simulink model "SF103A_MotorReferenceModel_v001B_MappedToEA4"  (R2013b)
settings: Solver=FixedStepDiscrete  StartTime=0.0  StopTime=10.0  RelTol=1e-3
InitFcn:
  | SF103A_MotorReferenceModel_v001X_Parameters;
undefined symbols (not defined in the file or in its folder): D_DTSCLMAX_ULS, D_DTSCLMIN_ULS, D_VECUMAX_VOLTS, D_VECUMIN_VOLTS, MtrCtrl_d_Ts_slow_s, MtrCtrl_e_KeNom_VpRadpS, MtrCtrl_e_RmNom_Ohm, MtrCtrl_k_deadtimeVScale_Uls, MtrCtrl_k_FeedbackControlDisable_Cnt, MtrCtrl_k_IdBoostGain_Uls, MtrCtrl_k_IdBoostVRThreshScl_Uls, MtrCtrl_k_IdqRefIminTol_Uls, MtrCtrl_k_IdqRefTrqTol_Uls, MtrCtrl_k_LdNom_Henry, MtrCtrl_k_LqNom_Henry, MtrCtrl_k_MtrCurrDaxMaxValScl_Per, MtrCtrl_k_MtrVoltDervFiltTimeConst_Sec, MtrCtrl_k_NoofPoles_Uls, MtrCtrl_k_VoltModeDynCompEnable_Cnt, MtrCtrl_t_IdBoostTrqCharSclY_Uls, MtrCtrl_t_IdBoostTrqCmdX_MtrNm, MtrCtrl_t_IdqRefDeltaPoints_Rad, MtrCtrl_t_Q13VltgSchedXTbl_MtrRadpS, MtrCtrl_t_Q13VltgSchedYTbl_Volt, MtrCtrl_t_Q24VltgSchedXTbl_MtrRadpS, MtrCtrl_t_Q24VltgSchedYTbl_Volt
undefined symbols (not defined in the file): MtrCtrl_k_MtrVelFiltFFKn_Hz
libraries: simulink x6
(part 1 of 2)
settings Model: Creator=SZJ6LD  LastModifiedBy=lzz0tm

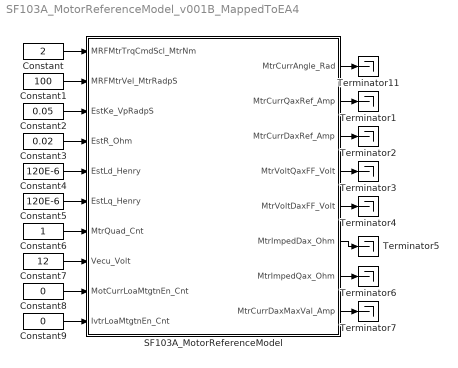
== system SF103A_MotorReferenceModel_v001B_MappedToEA4 ==
  Constant : Constant  Value=2
  Constant1 : Constant  Value=100
  Constant2 : Constant  Value=0.05
  Constant3 : Constant  Value=0.02
  Constant4 : Constant  Value=120E-6
  Constant5 : Constant  Value=120E-6
  Constant6 : Constant
  Constant7 : Constant  Value=12
  Constant8 : Constant  Value=0
  Constant9 : Constant  Value=0
  SF103A_MotorReferenceModel : Subsystem
      settings: AttributesFormatString=%<LibraryVersion>
  Terminator{1..7,11} (8 alike) : Terminator
  wires:
  SF103A_MotorReferenceModel/1(MtrCurrAngle_Rad) -> Terminator11/1
  SF103A_MotorReferenceModel/8(MtrCurrDaxMaxVal_Amp) -> Terminator7/1
  SF103A_MotorReferenceModel/7(MtrImpedQax_Ohm) -> Terminator6/1
  SF103A_MotorReferenceModel/6(MtrImpedDax_Ohm) -> Terminator5/1
  SF103A_MotorReferenceModel/5(MtrVoltDaxFF_Volt) -> Terminator4/1
  SF103A_MotorReferenceModel/4(MtrVoltQaxFF_Volt) -> Terminator3/1
  SF103A_MotorReferenceModel/3(MtrCurrDaxRef_Amp) -> Terminator2/1
  SF103A_MotorReferenceModel/2(MtrCurrQaxRef_Amp) -> Terminator1/1
  Constant/1 -> SF103A_MotorReferenceModel/1(MRFMtrTrqCmdScl_MtrNm)
  Constant1/1 -> SF103A_MotorReferenceModel/2(MRFMtrVel_MtrRadpS)
  Constant2/1 -> SF103A_MotorReferenceModel/3(EstKe_VpRadpS)
  Constant3/1 -> SF103A_MotorReferenceModel/4(EstR_Ohm)
  Constant4/1 -> SF103A_MotorReferenceModel/5(EstLd_Henry)
  Constant5/1 -> SF103A_MotorReferenceModel/6(EstLq_Henry)
  Constant6/1 -> SF103A_MotorReferenceModel/7(MtrQuad_Cnt)
  Constant7/1 -> SF103A_MotorReferenceModel/8(Vecu_Volt)
  Constant8/1 -> SF103A_MotorReferenceModel/9(MotCurrLoaMtgtnEn_Cnt)
  Constant9/1 -> SF103A_MotorReferenceModel/10(IvtrLoaMtgtnEn_Cnt)

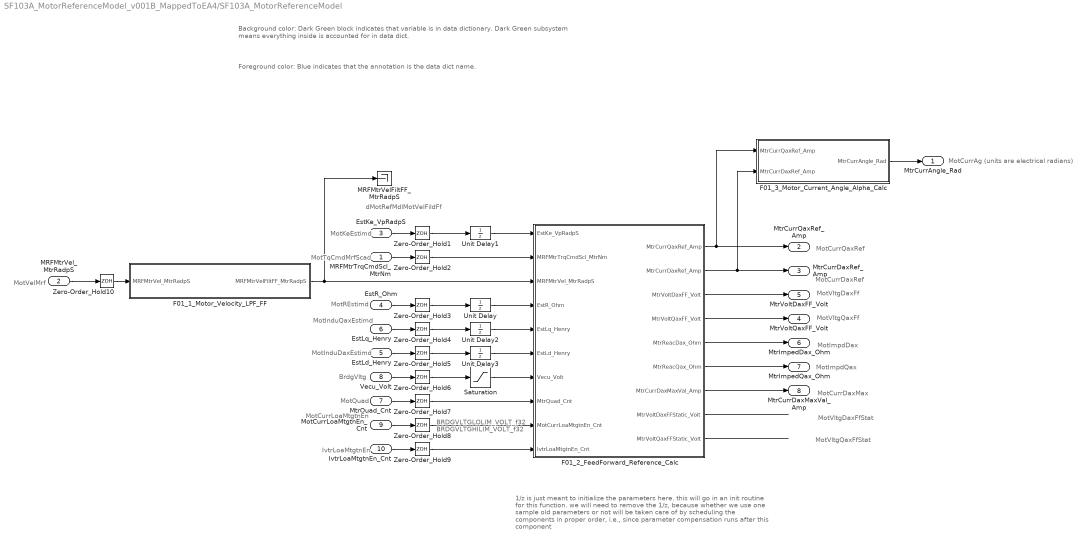
== system SF103A_MotorReferenceModel_v001B_MappedToEA4/SF103A_MotorReferenceModel ==
  note: MotVltgQaxFfStat
  note: MotVltgQaxFf
  note: MotVltgDaxFfStat
  note: MotVltgDaxFf
  note: MotImpdQax
  note: MotImpdDax
  note: MotCurrQaxRef
  note: MotCurrDaxRef
  note: MotCurrDaxMax
  note: MotCurrAg (units are electrical radians)
  note: dMotRefMdlMotVelFildFf
  note: BRDGVLTGLOLIM_VOLT_f32
      | BRDGVLTGHILIM_VOLT_f32
  note: 1/z is just meant to initialize the parameters here.
      | this will go in an init routine for this function.
      |
      | we will need to remove the 1/z, because whether we use one sample old
      | parameters or not will be taken care of by scheduling the components in
      | proper order, i.e., since parameter compensation runs after this component
  note: MotVelMrf
  note: MotTqCmdMrfScad
  note: MotREstimd
  note: MotQuad
  note: MotKeEstimd
  note: MotInduQaxEstimd
  note: MotInduDaxEstimd
  note: MotCurrLoaMtgtnEn
  note: IvtrLoaMtgtnEn
  note: BrdgVltg
  note: Background color:  Dark Green block indicates that variable is in data dictionary.
      |                                Dark Green subsystem means everything inside is accounted for in data dict.
  note: Foreground color: Blue indicates that the annotation is the data dict name.
  MRFMtrTrqCmdScl_MtrNm : Inport
  MRFMtrVel_MtrRadpS : Inport  Port=2
  EstKe_VpRadpS : Inport  Port=3
  EstR_Ohm : Inport  Port=4
  EstLd_Henry : Inport  Port=5
  EstLq_Henry : Inport  Port=6
  MtrQuad_Cnt : Inport  Port=7
  Vecu_Volt : Inport  Port=8
  MotCurrLoaMtgtnEn_Cnt : Inport  Port=9
  IvtrLoaMtgtnEn_Cnt : Inport  Port=10
  F01_1_Motor_Velocity_LPF_FF : Subsystem
  F01_2_FeedForward_Reference_Calc : Subsystem
  F01_3_Motor_Current_Angle_Alpha_Calc : Subsystem
  MRFMtrVelFiltFF_MtrRadpS : Terminator
  "Saturation  " : Saturate  UpperLimit=D_VECUMAX_VOLTS  LowerLimit=D_VECUMIN_VOLTS
      settings: AttributesFormatString=%<LowerLimit>\n%<UpperLimit>
  Unit Delay : UnitDelay  InitialCondition=MtrCtrl_e_RmNom_Ohm  SampleTime=MtrCtrl_d_Ts_slow_s
      settings: AttributesFormatString=Initial Value:\n%<X0>
  Unit Delay1 : UnitDelay  InitialCondition=MtrCtrl_e_KeNom_VpRadpS  SampleTime=MtrCtrl_d_Ts_slow_s
      settings: AttributesFormatString=Initial Value:\n%<X0>
  Unit Delay2 : UnitDelay  InitialCondition=MtrCtrl_k_LqNom_Henry  SampleTime=MtrCtrl_d_Ts_slow_s
      settings: AttributesFormatString=Initial Value:\n%<X0>
  Unit Delay3 : UnitDelay  InitialCondition=MtrCtrl_k_LdNom_Henry  SampleTime=MtrCtrl_d_Ts_slow_s
      settings: AttributesFormatString=Initial Value:\n%<X0>
  Zero-Order_Hold{1..10} (10 alike) : ZeroOrderHold  SampleTime=MtrCtrl_d_Ts_slow_s
  MtrCurrAngle_Rad : Outport
  MtrCurrQaxRef_Amp : Outport  Port=2
  MtrCurrDaxRef_Amp : Outport  Port=3
  MtrVoltQaxFF_Volt : Outport  Port=4
  MtrVoltDaxFF_Volt : Outport  Port=5
  MtrImpedDax_Ohm : Outport  Port=6
  MtrImpedQax_Ohm : Outport  Port=7
  MtrCurrDaxMaxVal_Amp : Outport  Port=8
  wires:
  F01_2_FeedForward_Reference_Calc/4(MtrVoltQaxFF_Volt) -> MtrVoltQaxFF_Volt/1
  F01_2_FeedForward_Reference_Calc/3(MtrVoltDaxFF_Volt) -> MtrVoltDaxFF_Volt/1
  F01_2_FeedForward_Reference_Calc/5(MtrReacDax_Ohm) -> MtrImpedDax_Ohm/1
  F01_2_FeedForward_Reference_Calc/6(MtrReacQax_Ohm) -> MtrImpedQax_Ohm/1
  MtrQuad_Cnt/1 -> Zero-Order_Hold7/1
  Vecu_Volt/1 -> Zero-Order_Hold6/1
  F01_3_Motor_Current_Angle_Alpha_Calc/1(MtrCurrAngle_Rad) -> MtrCurrAngle_Rad/1
  MRFMtrTrqCmdScl_MtrNm/1 -> Zero-Order_Hold2/1
  EstLq_Henry/1 -> Zero-Order_Hold4/1
  EstLd_Henry/1 -> Zero-Order_Hold5/1
  EstR_Ohm/1 -> Zero-Order_Hold3/1
  EstKe_VpRadpS/1 -> Zero-Order_Hold1/1
  F01_1_Motor_Velocity_LPF_FF/1(MRFMtrVelFiltFF_MtrRadpS) -> F01_2_FeedForward_Reference_Calc/3(MRFMtrVel_MtrRadpS), MRFMtrVelFiltFF_MtrRadpS/1
  MRFMtrVel_MtrRadpS/1 -> Zero-Order_Hold10/1
  F01_2_FeedForward_Reference_Calc/7(MtrCurrDaxMaxVal_Amp) -> MtrCurrDaxMaxVal_Amp/1
  F01_2_FeedForward_Reference_Calc/9(MtrVoltQaxFFStatic_Volt) -> ?
  F01_2_FeedForward_Reference_Calc/8(MtrVoltDaxFFStatic_Volt) -> ?
  MotCurrLoaMtgtnEn_Cnt/1 -> Zero-Order_Hold8/1
  F01_2_FeedForward_Reference_Calc/1(MtrCurrQaxRef_Amp) -> F01_3_Motor_Current_Angle_Alpha_Calc/1(MtrCurrQaxRef_Amp), MtrCurrQaxRef_Amp/1
  F01_2_FeedForward_Reference_Calc/2(MtrCurrDaxRef_Amp) -> F01_3_Motor_Current_Angle_Alpha_Calc/2(MtrCurrDaxRef_Amp), MtrCurrDaxRef_Amp/1
  Unit Delay/1 -> F01_2_FeedForward_Reference_Calc/4(EstR_Ohm)
  Unit Delay1/1 -> F01_2_FeedForward_Reference_Calc/1(EstKe_VpRadpS)
  Unit Delay2/1 -> F01_2_FeedForward_Reference_Calc/5(EstLq_Henry)
  Unit Delay3/1 -> F01_2_FeedForward_Reference_Calc/6(EstLd_Henry)
  Zero-Order_Hold10/1 -> F01_1_Motor_Velocity_LPF_FF/1(MRFMtrVel_MtrRadpS)
  Zero-Order_Hold1/1 -> Unit Delay1/1
  Zero-Order_Hold2/1 -> F01_2_FeedForward_Reference_Calc/2(MRFMtrTrqCmdScl_MtrNm)
  Zero-Order_Hold3/1 -> Unit Delay/1
  Zero-Order_Hold4/1 -> Unit Delay2/1
  Zero-Order_Hold5/1 -> Unit Delay3/1
  Zero-Order_Hold6/1 -> "Saturation  "/1
  Zero-Order_Hold7/1 -> F01_2_FeedForward_Reference_Calc/8(MtrQuad_Cnt)
  Zero-Order_Hold8/1 -> F01_2_FeedForward_Reference_Calc/9(MotCurrLoaMtgtnEn_Cnt)
  "Saturation  "/1 -> F01_2_FeedForward_Reference_Calc/7(Vecu_Volt)
  IvtrLoaMtgtnEn_Cnt/1 -> Zero-Order_Hold9/1
  Zero-Order_Hold9/1 -> F01_2_FeedForward_Reference_Calc/10(IvtrLoaMtgtnEn_Cnt)

== system SF103A_MotorReferenceModel_v001B_MappedToEA4/SF103A_MotorReferenceModel/F01_1_Motor_Velocity_LPF_FF ==
  note: MotRefMdlMotVelLpFiltFrq
  MRFMtrVel_MtrRadpS : Inport
  1LP1-CF Filter : Subsystem  mask{Ts=MtrCtrl_d_Ts_slow_s, Kn_Hz=MtrCtrl_k_MtrVelFiltFFKn_Hz, IC=0}
      mask prompts: Ts "Function Time Step (seconds)"; Kn_Hz "Cutoff Frequency in Hz"; IC "Initial Condition (Enineering Units)"
      mask init:
      | %Convert cutoff frequency from Hz into floating point "counts"
      | Kn_Cnt = 1-exp(-2*pi*Kn_Hz*Ts);
      | 
      | %Filter design document originally called this value Knum
      | Knum = Kn_Cnt;
      settings: AttributesFormatString=%<Kn_Hz>
      mask Display:
      | a = [2:0.1:5.2]';
      | b = sin(2*a);
      | c = 0.7*sin(25*a);
      | d = b+c;
      | e = vertcat(d, b);
      | plot(e);
  MRFMtrVelFiltFF_MtrRadpS : Outport
  wires:
  MRFMtrVel_MtrRadpS/1 -> 1LP1-CF Filter/1(In1)
  1LP1-CF Filter/1(Out) -> MRFMtrVelFiltFF_MtrRadpS/1

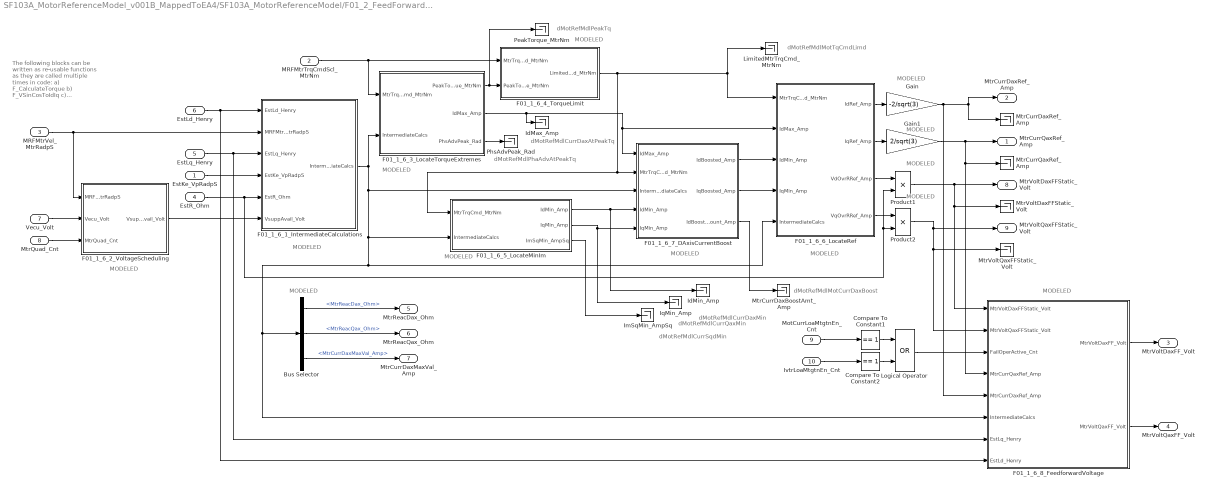
== system SF103A_MotorReferenceModel_v001B_MappedToEA4/SF103A_MotorReferenceModel/F01_2_FeedForward_Reference_Calc ==
  note: MODELED
  note: dMotRefMdlMotCurrDaxBoost
  note: dMotRefMdlCurrSqdMin
  note: dMotRefMdlCurrQaxMin
  note: dMotRefMdlCurrDaxMin
  note: dMotRefMdlCurrDaxAtPeakTq
  note: dMotRefMdlPhaAdvAtPeakTq
  note: dMotRefMdlPeakTq
  note: dMotRefMdlMotTqCmdLimd
  note: The following blocks can be written as re-usable functions
      | as they are called multiple times in code:
      | a) F_CalculateTorque
      | b)  F_VSinCosToIdIq
      | c) F_ParabolicInterpolation
      | d) F_CalcIqCommand
      | e) F_ImVSIdq
      | f) F_ItoV
      | g) F_VoltTest
  note: MODELED
  note: MODELED
  note: MODELED
  note: MODELED
  note: MODELED
  note: MODELED
  note: MODELED
  note: MODELED
  note: MODELED
  note: MODELED
  note: MODELED
  note: MODELED
  EstKe_VpRadpS : Inport
  MRFMtrTrqCmdScl_MtrNm : Inport  Port=2
  MRFMtrVel_MtrRadpS : Inport  Port=3
  EstR_Ohm : Inport  Port=4
  EstLq_Henry : Inport  Port=5
  EstLd_Henry : Inport  Port=6
  Vecu_Volt : Inport  Port=7
  MtrQuad_Cnt : Inport  Port=8
  MotCurrLoaMtgtnEn_Cnt : Inport  Port=9
  IvtrLoaMtgtnEn_Cnt : Inport  Port=10
  Bus Selector : BusSelector  OutputSignals=MtrReacDax_Ohm,MtrReacQax_Ohm,MtrCurrDaxMaxVal_Amp
  Compare To Constant1 : simulink/Logic and Bit Operations/Compare To Constant  relop===  const=1  OutDataTypeStr=uint8
  Compare To Constant2 : simulink/Logic and Bit Operations/Compare To Constant  relop===  const=1  OutDataTypeStr=uint8
  F01_1_6_1_IntermediateCalculations : Subsystem
  F01_1_6_2_VoltageScheduling : Subsystem
  F01_1_6_3_LocateTorqueExtremes : Subsystem
  F01_1_6_4_TorqueLimit : Subsystem
  F01_1_6_5_LocateMinIm : Subsystem
  F01_1_6_6_LocateRef : Subsystem
  F01_1_6_7_DAxisCurrentBoost : Subsystem
  F01_1_6_8_FeedforwardVoltage : Subsystem
  Gain : Gain  Gain=-2/sqrt(3)
  Gain1 : Gain  Gain=2/sqrt(3)
  IdMax_Amp : Terminator
  IdMin_Amp : Terminator
  ImSqMin_AmpSq : Terminator
  IqMin_Amp : Terminator
  "LimitedMtrTrqCmd_MtrNm " : Terminator
  Logical Operator : Logic  Operator=OR  AllPortsSameDT=off  OutDataTypeStr=boolean
  MtrCurrDaxBoostAmt_Amp : Terminator
  "MtrCurrDaxRef_Amp " : Terminator
  "MtrCurrQaxRef_Amp " : Terminator
  "MtrVoltDaxFFStatic_Volt " : Terminator
  "MtrVoltQaxFFStatic_Volt " : Terminator
  PeakTorque_MtrNm : Terminator
  PhsAdvPeak_Rad : Terminator
  Product1 : Product  RndMeth=Zero
  Product2 : Product  RndMeth=Zero
  MtrCurrQaxRef_Amp : Outport
  MtrCurrDaxRef_Amp : Outport  Port=2
  MtrVoltDaxFF_Volt : Outport  Port=3
  MtrVoltQaxFF_Volt : Outport  Port=4
  MtrReacDax_Ohm : Outport  Port=5
  MtrReacQax_Ohm : Outport  Port=6
  MtrCurrDaxMaxVal_Amp : Outport  Port=7
  MtrVoltDaxFFStatic_Volt : Outport  Port=8
  MtrVoltQaxFFStatic_Volt : Outport  Port=9
  wires:
  Gain/1 -> F01_1_6_8_FeedforwardVoltage/5(MtrCurrDaxRef_Amp), MtrCurrDaxRef_Amp/1, "MtrCurrDaxRef_Amp "/1
  Product2/1 -> F01_1_6_8_FeedforwardVoltage/2(MtrVoltQaxFFStatic_Volt), "MtrVoltQaxFFStatic_Volt "/1, MtrVoltQaxFFStatic_Volt/1
  Product1/1 -> F01_1_6_8_FeedforwardVoltage/1(MtrVoltDaxFFStatic_Volt), "MtrVoltDaxFFStatic_Volt "/1, MtrVoltDaxFFStatic_Volt/1
  Gain1/1 -> F01_1_6_8_FeedforwardVoltage/4(MtrCurrQaxRef_Amp), "MtrCurrQaxRef_Amp "/1, MtrCurrQaxRef_Amp/1
  F01_1_6_8_FeedforwardVoltage/2(MtrVoltQaxFF_Volt) -> MtrVoltQaxFF_Volt/1
  F01_1_6_8_FeedforwardVoltage/1(MtrVoltDaxFF_Volt) -> MtrVoltDaxFF_Volt/1
  Bus Selector/1 -> MtrReacDax_Ohm/1  "<MtrReacDax_Ohm>"
  Bus Selector/2 -> MtrReacQax_Ohm/1  "<MtrReacQax_Ohm>"
  F01_1_6_7_DAxisCurrentBoost/3(IdBoostAmount_Amp) -> MtrCurrDaxBoostAmt_Amp/1
  F01_1_6_7_DAxisCurrentBoost/2(IqBoosted_Amp) -> F01_1_6_6_LocateRef/4(IqMin_Amp)
  F01_1_6_7_DAxisCurrentBoost/1(IdBoosted_Amp) -> F01_1_6_6_LocateRef/3(IdMin_Amp)
  MtrQuad_Cnt/1 -> F01_1_6_2_VoltageScheduling/3(MtrQuad_Cnt)
  Vecu_Volt/1 -> F01_1_6_2_VoltageScheduling/2(Vecu_Volt)
  F01_1_6_2_VoltageScheduling/1(VsuppAvail_Volt) -> F01_1_6_1_IntermediateCalculations/6(VsuppAvail_Volt)
  F01_1_6_6_LocateRef/4(VqOvrRRef_Amp) -> Product2/1
  F01_1_6_6_LocateRef/3(VdOvrRRef_Amp) -> Product1/1
  F01_1_6_6_LocateRef/2(IqRef_Amp) -> Gain1/1
  F01_1_6_6_LocateRef/1(IdRef_Amp) -> Gain/1
  F01_1_6_5_LocateMinIm/3(ImSqMin_AmpSq) -> ImSqMin_AmpSq/1
  F01_1_6_3_LocateTorqueExtremes/3(PhsAdvPeak_Rad) -> PhsAdvPeak_Rad/1
  F01_1_6_5_LocateMinIm/2(IqMin_Amp) -> F01_1_6_7_DAxisCurrentBoost/5(IqMin_Amp), IqMin_Amp/1
  F01_1_6_5_LocateMinIm/1(IdMin_Amp) -> F01_1_6_7_DAxisCurrentBoost/4(IdMin_Amp), IdMin_Amp/1
  F01_1_6_3_LocateTorqueExtremes/2(IdMax_Amp) -> F01_1_6_7_DAxisCurrentBoost/1(IdMax_Amp), F01_1_6_6_LocateRef/2(IdMax_Amp), IdMax_Amp/1
  MRFMtrTrqCmdScl_MtrNm/1 -> F01_1_6_3_LocateTorqueExtremes/1(MtrTrqCmd_MtrNm), F01_1_6_4_TorqueLimit/1(MtrTrqCmd_MtrNm)
  F01_1_6_3_LocateTorqueExtremes/1(PeakTorque_MtrNm) -> PeakTorque_MtrNm/1, F01_1_6_4_TorqueLimit/2(PeakTorque_MtrNm)
  EstR_Ohm/1 -> Product2/2, Product1/2, F01_1_6_1_IntermediateCalculations/5(EstR_Ohm)
  EstKe_VpRadpS/1 -> F01_1_6_1_IntermediateCalculations/4(EstKe_VpRadpS)
  MRFMtrVel_MtrRadpS/1 -> F01_1_6_2_VoltageScheduling/1(MRFMtrVel_MtrRadpS), F01_1_6_1_IntermediateCalculations/2(MRFMtrVel_MtrRadpS)
  EstLd_Henry/1 -> F01_1_6_1_IntermediateCalculations/1(EstLd_Henry), F01_1_6_8_FeedforwardVoltage/8(EstLd_Henry)
  F01_1_6_1_IntermediateCalculations/1(IntermediateCalcs) -> F01_1_6_7_DAxisCurrentBoost/3(IntermediateCalcs), F01_1_6_5_LocateMinIm/2(IntermediateCalcs), F01_1_6_6_LocateRef/5(IntermediateCalcs), F01_1_6_8_FeedforwardVoltage/6(IntermediateCalcs), Bus Selector/1, F01_1_6_3_LocateTorqueExtremes/2(IntermediateCalcs)
  F01_1_6_4_TorqueLimit/1(LimitedMtrTrqCmd_MtrNm) -> F01_1_6_5_LocateMinIm/1(MtrTrqCmd_MtrNm), F01_1_6_7_DAxisCurrentBoost/2(MtrTrqCmd_MtrNm), "LimitedMtrTrqCmd_MtrNm "/1, F01_1_6_6_LocateRef/1(MtrTrqCmd_MtrNm)
  Compare To Constant1/1 -> Logical Operator/1
  EstLq_Henry/1 -> F01_1_6_8_FeedforwardVoltage/7(EstLq_Henry), F01_1_6_1_IntermediateCalculations/3(EstLq_Henry)
  Bus Selector/3 -> MtrCurrDaxMaxVal_Amp/1  "<MtrCurrDaxMaxVal_Amp>"
  Compare To Constant2/1 -> Logical Operator/2
  Logical Operator/1 -> F01_1_6_8_FeedforwardVoltage/3(FailOperActive_Cnt)
  MotCurrLoaMtgtnEn_Cnt/1 -> Compare To Constant1/1
  IvtrLoaMtgtnEn_Cnt/1 -> Compare To Constant2/1

== system SF103A_MotorReferenceModel_v001B_MappedToEA4/SF103A_MotorReferenceModel/F01_3_Motor_Current_Angle_Alpha_Calc ==
  MtrCurrQaxRef_Amp : Inport
  MtrCurrDaxRef_Amp : Inport  Port=2
  atan2 : Trigonometry  Operator=atan2
  MtrCurrAngle_Rad : Outport
  wires:
  MtrCurrQaxRef_Amp/1 -> atan2/2
  MtrCurrDaxRef_Amp/1 -> atan2/1
  atan2/1 -> MtrCurrAngle_Rad/1

== system SF103A_MotorReferenceModel_v001B_MappedToEA4/SF103A_MotorReferenceModel/F01_1_Motor_Velocity_LPF_FF/1LP1-CF Filter ==
  note: Filter layout from spreadsheet
  note: This Subsystem represents a type 1LP1-CF Low-Pass filter with floating point math. Layout and nomenclature taken from Design Document authored by Mark Colosky.
  note: REVISIONS
      |   Feb 13, 2012.  Date created.
      |   Feb 17, 2012.  Conversion from Hz to Knum moved to Initialization tab of mask dialog box.
      |   Feb 20, 2012.  Parameterized 1/z block Initial Condition instead of hard-coded = 0.
  In1 : Inport
  Constant : Constant  Value=Knum  SampleTime=Ts
  Integer Delay : Delay  DelayLength=1  InitialCondition=IC  SampleTime=Ts
  Product1 : Product  RndMeth=Zero
  Sum : Sum  Inputs=|+-
  Sum1 : Sum  Inputs=|++
  Out : Outport
  wires:
  Sum1/1 -> Out/1, Integer Delay/1  "e"
  In1/1 -> Sum/1  "Unfiltered_Signal"
  Integer Delay/1 -> Sum/2, Sum1/2  "f"
  Product1/1 -> Sum1/1  "d"
  Constant/1 -> Product1/1
  Sum/1 -> Product1/2  "c"

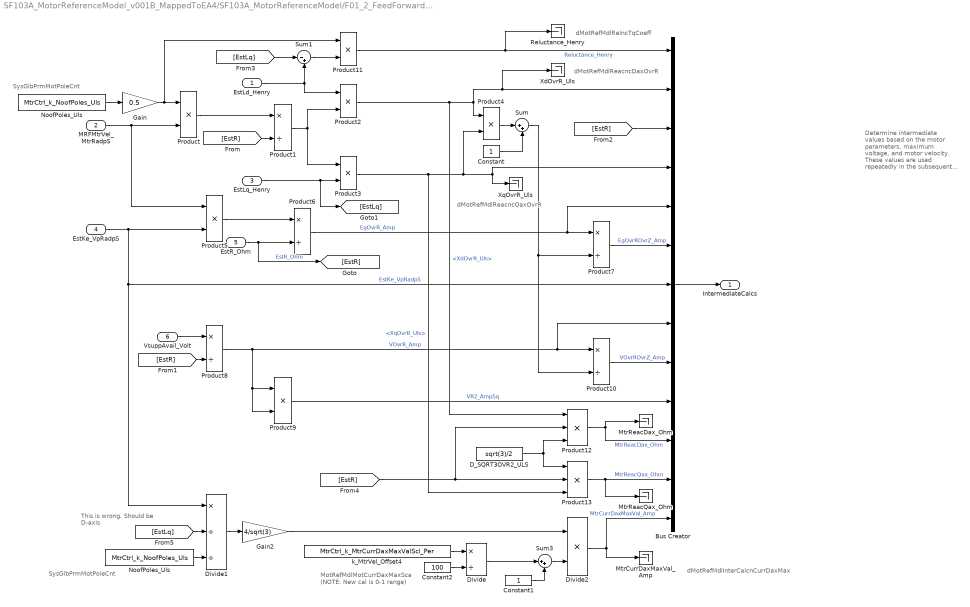
== system SF103A_MotorReferenceModel_v001B_MappedToEA4/SF103A_MotorReferenceModel/F01_2_FeedForward_Reference_Calc/F01_1_6_1_IntermediateCalculations ==
  note: This is wrong.
      | Should be D-axis
  note: MotRefMdlMotCurrDaxMaxSca
      | (NOTE:  New cal is 0-1 range)
  note: SysGlbPrmMotPoleCnt
  note: dMotRefMdlReacncDaxOvrR
  note: dMotRefMdlRelncTqCoeff
  note: dMotRefMdlInterCalcnCurrDaxMax
  note: Determine intermediate values based on the motor parameters, maximum voltage, and motor velocity.
      | These values are used repeatedly in the subsequent iterative solutions and performing these calculations once
      | in advance decreases computation time and reduces the possibility of introducing error.
  note: dMotRefMdlReacncQaxOvrR
  note: SysGlbPrmMotPoleCnt
  EstLd_Henry : Inport
  MRFMtrVel_MtrRadpS : Inport  Port=2
  EstLq_Henry : Inport  Port=3
  EstKe_VpRadpS : Inport  Port=4
  EstR_Ohm : Inport  Port=5
  VsuppAvail_Volt : Inport  Port=6
  Bus Creator : BusCreator  Inputs=13
  Constant : Constant
  Constant1 : Constant  SampleTime=MtrCtrl_d_Ts_slow_s
  Constant2 : Constant  Value=100  SampleTime=MtrCtrl_d_Ts_slow_s
  D_SQRT3OVR2_ULS : Constant  Value=sqrt(3)/2  SampleTime=MtrCtrl_d_Ts_slow_s
  Divide : Product  Inputs=*/
  Divide1 : Product  Inputs=*//
  Divide2 : Product
  Gain : Gain  Gain=0.5  SampleTime=MtrCtrl_d_Ts_slow_s
  Gain2 : Gain  Gain=4/sqrt(3)  SampleTime=MtrCtrl_d_Ts_slow_s
  "MtrCurrDaxMaxVal_Amp  " : Terminator
  "MtrReacDax_Ohm   " : Terminator
  "MtrReacQax_Ohm  " : Terminator
  NoofPoles_Uls : Constant  Value=MtrCtrl_k_NoofPoles_Uls
  "NoofPoles_Uls " : Constant  Value=MtrCtrl_k_NoofPoles_Uls
  Product : Product  SampleTime=MtrCtrl_d_Ts_slow_s  RndMeth=Zero
  Product1 : Product  Inputs=*/  RndMeth=Zero
  Product10 : Product  Inputs=*/  SampleTime=MtrCtrl_d_Ts_slow_s  RndMeth=Zero
  Product{2..4,11} (4 alike) : Product  RndMeth=Zero
  Product12 : Product  Inputs=3  RndMeth=Zero
  Product13 : Product  Inputs=3  RndMeth=Zero
  Product5 : Product  SampleTime=MtrCtrl_d_Ts_slow_s  RndMeth=Zero
  Product6 : Product  Inputs=*/  RndMeth=Zero
  Product7 : Product  Inputs=*/  SampleTime=MtrCtrl_d_Ts_slow_s  RndMeth=Zero
  Product8 : Product  Inputs=*/  SampleTime=MtrCtrl_d_Ts_slow_s  RndMeth=Zero
  Product9 : Product  SampleTime=MtrCtrl_d_Ts_slow_s  RndMeth=Zero
  Reluctance_Henry : Terminator
  Sum : Sum  Inputs=|++
  Sum1 : Sum  Inputs=|-+
  Sum3 : Sum  Inputs=|++
  XdOvrR_Uls : Terminator
  XqOvrR_Uls : Terminator
  k_MtrVel_Offset4 : Constant  Value=MtrCtrl_k_MtrCurrDaxMaxValScl_Per  SampleTime=MtrCtrl_d_Ts_slow_s
  IntermediateCalcs : Outport
  wires:
  VsuppAvail_Volt/1 -> Product8/1
  Bus Creator/1 -> IntermediateCalcs/1
  NoofPoles_Uls/1 -> Gain/1
  Product10/1 -> Bus Creator/9  "VOvrROvrZ_Amp"
  Product11/1 -> Bus Creator/1, Reluctance_Henry/1  "Reluctance_Henry"
  Sum1/1 -> Product11/2
  [EstLq] -> Sum1/1
  [EstR] -> Bus Creator/3
  Product9/1 -> Bus Creator/10  "VR2_AmpSq"
  Product8/1 -> Bus Creator/8, Product10/1, Product9/2, Product9/1  "VOvrR_Amp"
  [EstR] -> Product8/2
  Product7/1 -> Bus Creator/6  "EgOvrROvrZ_Amp"
  Product6/1 -> Bus Creator/5, Product7/1  "EgOvrR_Amp"
  [EstR] -> Product1/2
  EstR_Ohm/1 -> Product6/2, [EstR]  "EstR_Ohm"
  Product5/1 -> Product6/1
  EstKe_VpRadpS/1 -> Product5/2, Divide1/1, Bus Creator/7  "EstKe_VpRadpS"
  Sum/1 -> Product10/2, Product7/2
  Constant/1 -> Sum/2
  Product4/1 -> Sum/1
  EstLq_Henry/1 -> Product3/2, [EstLq]
  EstLd_Henry/1 -> Sum1/2, Product2/1
  Product1/1 -> Product3/1, Product2/2
  Product/1 -> Product1/1
  MRFMtrVel_MtrRadpS/1 -> Product5/1, Product/2
  Gain/1 -> Product11/1, Product/1
  D_SQRT3OVR2_ULS/1 -> Product12/3, Product13/1
  Product3/1 -> Product13/3, XqOvrR_Uls/1, Bus Creator/4, Product4/2  "<XqOvrR_Uls>"
  [EstR] -> Product12/2, Product13/2
  Product13/1 -> Bus Creator/12, "MtrReacQax_Ohm  "/1  "MtrReacQax_Ohm"
  Product12/1 -> "MtrReacDax_Ohm   "/1, Bus Creator/11  "MtrReacDax_Ohm"
  Product2/1 -> Product12/1, XdOvrR_Uls/1, Bus Creator/2, Product4/1  "<XdOvrR_Uls>"
  "NoofPoles_Uls "/1 -> Divide1/3
  Divide1/1 -> Gain2/1
  Gain2/1 -> Divide2/1
  Constant1/1 -> Sum3/2
  Divide/1 -> Sum3/1
  k_MtrVel_Offset4/1 -> Divide/1
  Constant2/1 -> Divide/2
  Sum3/1 -> Divide2/2
  Divide2/1 -> Bus Creator/13, "MtrCurrDaxMaxVal_Amp  "/1  "MtrCurrDaxMaxVal_Amp"
  [EstLq] -> Divide1/2

== system SF103A_MotorReferenceModel_v001B_MappedToEA4/SF103A_MotorReferenceModel/F01_2_FeedForward_Reference_Calc/F01_1_6_2_VoltageScheduling ==
  note: IVTRDEADTIBRDGVLTGSCALOLIM_ULS_F32
      | IVTRDEADTIBRDGVLTGSCAHILIM_ULS_F32
  note: MotRefMdlIvtrDeadTiBrdgVltgSca
  note: MotRefMdlQ13VltgSdlXTbl
      | MotRefMdlQ13VltgSdlYTbl
  note: MotRefMdlQ24VltgSdlXTbl
      | MotRefMdlQ24VltgSdlYTbl
  MRFMtrVel_MtrRadpS : Inport
  Vecu_Volt : Inport  Port=2
  MtrQuad_Cnt : Inport  Port=3
  Abs : Abs  SampleTime=MtrCtrl_d_Ts_slow_s
  Compare To Constant : simulink/Logic and Bit Operations/Compare To Constant  relop===  const=3.0  OutDataTypeStr=uint8
  Compare To Constant1 : simulink/Logic and Bit Operations/Compare To Constant  relop===  const=1  OutDataTypeStr=uint8
  Logical Operator : Logic  Operator=OR  AllPortsSameDT=off  OutDataTypeStr=boolean
  Lookup Table : Lookup  InputValues=MtrCtrl_t_Q13VltgSchedXTbl_MtrRadpS  Table=MtrCtrl_t_Q13VltgSchedYTbl_Volt  LookUpMeth=Interpolation-Use End Values
      settings: AttributesFormatString=%<InputValues>\n%<Table>
  Lookup Table1 : Lookup  InputValues=MtrCtrl_t_Q24VltgSchedXTbl_MtrRadpS  Table=MtrCtrl_t_Q24VltgSchedYTbl_Volt  LookUpMeth=Interpolation-Use End Values
      settings: AttributesFormatString=%<InputValues>\n%<Table>
  Product : Product  RndMeth=Zero
  "Saturation  " : Saturate  UpperLimit=D_DTSCLMAX_ULS  LowerLimit=D_DTSCLMIN_ULS
      settings: AttributesFormatString=%<LowerLimit>\n%<UpperLimit>
  Sum : Sum  Inputs=|+-
  Switch : Switch  Criteria=u2 > Threshold
  k_deadtimeVScale : Constant  Value=MtrCtrl_k_deadtimeVScale_Uls  SampleTime=MtrCtrl_d_Ts_slow_s
  VsuppAvail_Volt : Outport
  wires:
  Sum/1 -> VsuppAvail_Volt/1
  Switch/1 -> Sum/2
  Lookup Table1/1 -> Switch/3
  Lookup Table/1 -> Switch/1
  Logical Operator/1 -> Switch/2
  MtrQuad_Cnt/1 -> Compare To Constant1/1, Compare To Constant/1
  Compare To Constant1/1 -> Logical Operator/2
  Compare To Constant/1 -> Logical Operator/1
  Product/1 -> Sum/1
  k_deadtimeVScale/1 -> "Saturation  "/1
  Vecu_Volt/1 -> Product/1
  Abs/1 -> Lookup Table1/1, Lookup Table/1
  MRFMtrVel_MtrRadpS/1 -> Abs/1
  "Saturation  "/1 -> Product/2

== system SF103A_MotorReferenceModel_v001B_MappedToEA4/SF103A_MotorReferenceModel/F01_2_FeedForward_Reference_Calc/F01_1_6_3_LocateTorqueExtremes ==
  note: Determine the maximum possible torque and the direct axis current that corresponds to that current given the Intermediate calculation values
      |  and the sign of the torque command.  In order to do this, a series of search brackets are created by rotating the voltage vector completely around
      |  a circle in a finite number of steps.  Then the bracket array is searched for the maximum. If the resulting brackets include an angle of zero, the
      | brackets are adjusted to wrap the angle and avoid a discontinuity at zero. Finally, iterative parabolic interpolation is used to refine the
      | location of the maximum.
  note: MODELED
      | (Init runnable)
  note: MODELED
  note: MODELED
  note: MODELED
  note: MODELED
  MtrTrqCmd_MtrNm : Inport
  IntermediateCalcs : Inport  Port=2
  F01_1_6_3_1_FillBracketArrays : Subsystem
  F01_1_6_3_2_FindPeakTorques : Subsystem
  F01_1_6_3_3_ChooseDeltaBrackets : Subsystem
  F01_1_6_3_4_WrapBracketAngles : Subsystem
  F01_1_6_3_5_InterpolatePeakTorque : Subsystem
  PeakTorque_MtrNm : Outport
  IdMax_Amp : Outport  Port=2
  PhsAdvPeak_Rad : Outport  Port=3
  wires:
  MtrTrqCmd_MtrNm/1 -> F01_1_6_3_2_FindPeakTorques/2(MtrTrqCmd_MtrNm)
  F01_1_6_3_5_InterpolatePeakTorque/3(PhsAdvPeak_Rad) -> PhsAdvPeak_Rad/1
  F01_1_6_3_5_InterpolatePeakTorque/2(IdMax_Amp) -> IdMax_Amp/1
  F01_1_6_3_5_InterpolatePeakTorque/1(PeakTorque_MtrNm) -> PeakTorque_MtrNm/1
  F01_1_6_3_4_WrapBracketAngles/1(Points) -> F01_1_6_3_5_InterpolatePeakTorque/1(Points)
  F01_1_6_3_2_FindPeakTorques/1(PeakTrqIndex) -> F01_1_6_3_4_WrapBracketAngles/2(Index)
  F01_1_6_3_3_ChooseDeltaBrackets/1(Brackets) -> F01_1_6_3_4_WrapBracketAngles/1(Brackets), F01_1_6_3_2_FindPeakTorques/1(Brackets)
  F01_1_6_3_1_FillBracketArrays/1(BracketArray) -> F01_1_6_3_3_ChooseDeltaBrackets/1(BracketArray)
  IntermediateCalcs/1 -> F01_1_6_3_5_InterpolatePeakTorque/2(IntermediateCalcs), F01_1_6_3_3_ChooseDeltaBrackets/2(IntermediateCalcs)

== system SF103A_MotorReferenceModel_v001B_MappedToEA4/SF103A_MotorReferenceModel/F01_2_FeedForward_Reference_Calc/F01_1_6_4_TorqueLimit ==
  note: Limit the torque command to less than or equal to the value found in
      |  Locate Torque Extremes  to avoid searching for impossible solutions
  MtrTrqCmd_MtrNm : Inport
  PeakTorque_MtrNm : Inport  Port=2
  Sum : Sum  Inputs=|-+
  Sum1 : Sum  Inputs=+-|
  Switch : Switch
  Switch1 : Switch  Criteria=u2 > Threshold
  Switch2 : Switch
  LimitedMtrTrqCmd_MtrNm : Outport
  wires:
  Switch2/1 -> Switch/3
  Switch1/1 -> Switch/1
  Sum1/1 -> Switch2/2
  Sum/1 -> Switch1/2
  PeakTorque_MtrNm/1 -> Switch1/1, Sum/1, Switch2/3, Sum1/2
  Switch/1 -> LimitedMtrTrqCmd_MtrNm/1
  MtrTrqCmd_MtrNm/1 -> Switch2/1, Sum1/1, Switch1/3, Sum/2, Switch/2

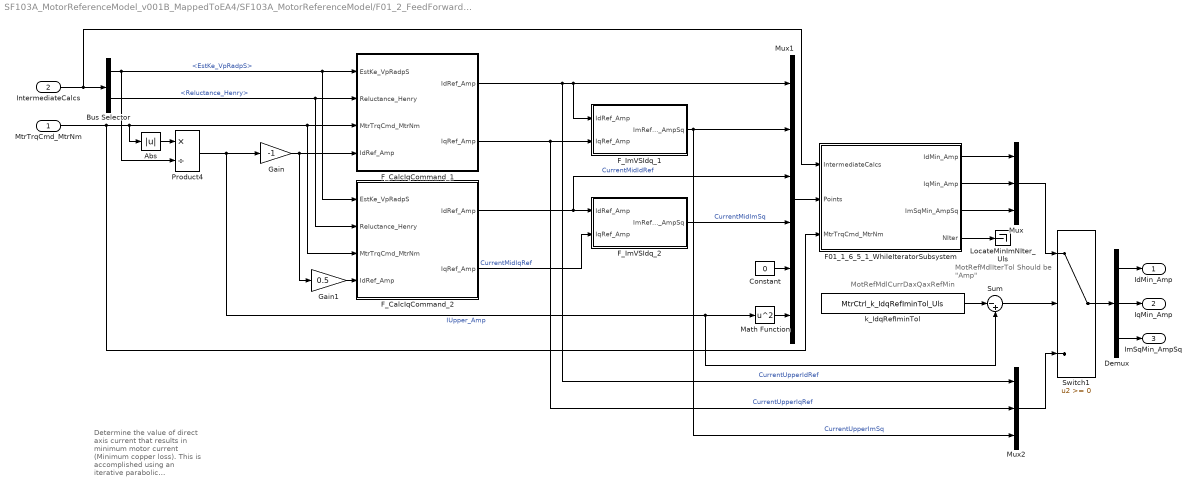
== system SF103A_MotorReferenceModel_v001B_MappedToEA4/SF103A_MotorReferenceModel/F01_2_FeedForward_Reference_Calc/F01_1_6_5_LocateMinIm ==
  note: MotRefMdlIterTol
      | Should be "Amp"
  note: MotRefMdlCurrDaxQaxRefMin
  note: Determine the value of direct axis current that results in minimum motor current (Minimum copper loss).
      | This is accomplished using an iterative parabolic interpolation. The triple of points used to initialize the
      | interpolation include:
      | a.	Direct axis current equal to zero
      | b.	Direct axis current equal to torque command divided by motor constant
      | c.	Direct axis current equal to one half of point b.
  MtrTrqCmd_MtrNm : Inport
  IntermediateCalcs : Inport  Port=2
  Abs : Abs
  Bus Selector : BusSelector  OutputSignals=EstKe_VpRadpS,Reluctance_Henry
  Constant : Constant  Value=0
  Demux : Demux  Outputs=3
  F01_1_6_5_1_WhileIteratorSubsystem : Subsystem  TreatAsAtomicUnit=on
  F_CalcIqCommand_1 : Subsystem
  F_CalcIqCommand_2 : Subsystem
  F_ImVSIdq_1 : Subsystem
  F_ImVSIdq_2 : Subsystem
  Gain : Gain  Gain=-1
  Gain1 : Gain  Gain=0.5
  LocateMinImNIter_Uls : Terminator
  Math Function : Math  Operator=square  SaturateOnIntegerOverflow=on
  Mux : Mux  Inputs=3
  Mux1 : Mux  Inputs=6
  Mux2 : Mux  Inputs=3
  Product4 : Product  Inputs=*/  RndMeth=Zero
  Sum : Sum  Inputs=|-+
  Switch1 : Switch
  k_IdqRefIminTol : Constant  Value=MtrCtrl_k_IdqRefIminTol_Uls
  IdMin_Amp : Outport
  IqMin_Amp : Outport  Port=2
  ImSqMin_AmpSq : Outport  Port=3
  wires:
  F01_1_6_5_1_WhileIteratorSubsystem/4(NIter) -> LocateMinImNIter_Uls/1
  Demux/2 -> IqMin_Amp/1
  Demux/1 -> IdMin_Amp/1
  F01_1_6_5_1_WhileIteratorSubsystem/2(IqMin_Amp) -> Mux/2
  F01_1_6_5_1_WhileIteratorSubsystem/1(IdMin_Amp) -> Mux/1
  Demux/3 -> ImSqMin_AmpSq/1
  Switch1/1 -> Demux/1
  Mux/1 -> Switch1/1
  Mux2/1 -> Switch1/3
  F01_1_6_5_1_WhileIteratorSubsystem/3(ImSqMin_AmpSq) -> Mux/3
  Sum/1 -> Switch1/2
  k_IdqRefIminTol/1 -> Sum/1
  Mux1/1 -> F01_1_6_5_1_WhileIteratorSubsystem/2(Points)
  IntermediateCalcs/1 -> F01_1_6_5_1_WhileIteratorSubsystem/1(IntermediateCalcs), Bus Selector/1
  Math Function/1 -> Mux1/6
  Constant/1 -> Mux1/5
  F_ImVSIdq_2/1(ImRefSq_AmpSq) -> Mux1/4  "CurrentMidImSq"
  F_CalcIqCommand_2/1(IdRef_Amp) -> F_ImVSIdq_2/1(IdRef_Amp), Mux1/3  "CurrentMidIdRef"
  F_CalcIqCommand_2/2(IqRef_Amp) -> F_ImVSIdq_2/2(IqRef_Amp)  "CurrentMidIqRef"
  Gain1/1 -> F_CalcIqCommand_2/4("IdRef_Amp ")
  F_ImVSIdq_1/1(ImRefSq_AmpSq) -> Mux2/3, Mux1/2  "CurrentUpperImSq"
  F_CalcIqCommand_1/1(IdRef_Amp) -> Mux2/1, F_ImVSIdq_1/1(IdRef_Amp), Mux1/1  "CurrentUpperIdRef"
  Gain/1 -> F_CalcIqCommand_1/4("IdRef_Amp "), Gain1/1
  Product4/1 -> Gain/1, Sum/2, Math Function/1  "IUpper_Amp"
  Abs/1 -> Product4/1
  MtrTrqCmd_MtrNm/1 -> F01_1_6_5_1_WhileIteratorSubsystem/3(MtrTrqCmd_MtrNm), F_CalcIqCommand_1/3(MtrTrqCmd_MtrNm), F_CalcIqCommand_2/3(MtrTrqCmd_MtrNm), Abs/1
  F_CalcIqCommand_1/2(IqRef_Amp) -> F_ImVSIdq_1/2(IqRef_Amp), Mux2/2  "CurrentUpperIqRef"
  Bus Selector/2 -> F_CalcIqCommand_1/2(Reluctance_Henry), F_CalcIqCommand_2/2(Reluctance_Henry)  "<Reluctance_Henry>"
  Bus Selector/1 -> F_CalcIqCommand_1/1(EstKe_VpRadpS), F_CalcIqCommand_2/1(EstKe_VpRadpS), Product4/2  "<EstKe_VpRadpS>"

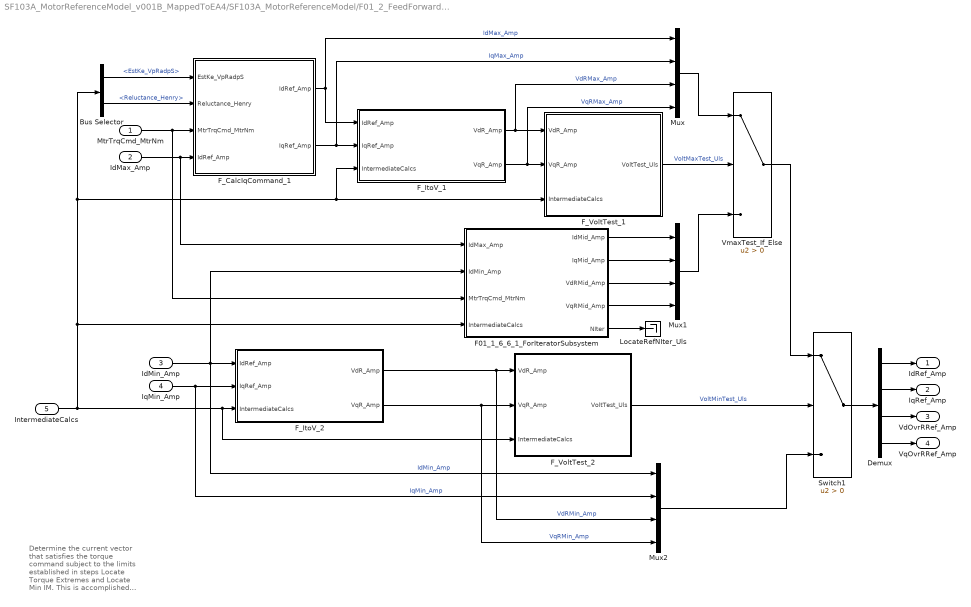
== system SF103A_MotorReferenceModel_v001B_MappedToEA4/SF103A_MotorReferenceModel/F01_2_FeedForward_Reference_Calc/F01_1_6_6_LocateRef ==
  note: Determine the current vector that satisfies the torque command subject to the limits established in steps Locate Torque
      | Extremes and Locate Min IM.
      | This is accomplished using an interval bisection search using the direct axis currents from steps Locate Torque Extremes
      | and Locate Min IM as brackets. If the current established in step Locate Min IM satisfies the torque command, The current
      | vector determined in that step is used and the search is not performed. If the current established in step Locate Torque
      | Extremes is not enough to satisfy the torque command, then the current vector established in that step is used and the search
      | is not performed. In all cases, the equations used in establishing the brackets and within the search loop yield the current
      | vector in Cartesian coordinates and also the voltage vector in Cartesian coordinates as an intermediate result.
  MtrTrqCmd_MtrNm : Inport
  IdMax_Amp : Inport  Port=2
  IdMin_Amp : Inport  Port=3
  IqMin_Amp : Inport  Port=4
  IntermediateCalcs : Inport  Port=5
  Bus Selector : BusSelector  OutputSignals=EstKe_VpRadpS,Reluctance_Henry
  Demux : Demux
  F01_1_6_6_1_ForIteratorSubsystem : Subsystem  TreatAsAtomicUnit=on
  F_CalcIqCommand_1 : Subsystem
  "F_ItoV_1 " : Subsystem
  F_ItoV_2 : Subsystem
  F_VoltTest_1 : Subsystem
  F_VoltTest_2 : Subsystem
  LocateRefNIter_Uls : Terminator
  Mux : Mux
  Mux1 : Mux
  Mux2 : Mux
  Switch1 : Switch  Criteria=u2 > Threshold  SampleTime=MtrCtrl_d_Ts_slow_s
  VmaxTest_If_Else : Switch  Criteria=u2 > Threshold  SampleTime=MtrCtrl_d_Ts_slow_s
  IdRef_Amp : Outport
  IqRef_Amp : Outport  Port=2
  VdOvrRRef_Amp : Outport  Port=3
  VqOvrRRef_Amp : Outport  Port=4
  wires:
  F01_1_6_6_1_ForIteratorSubsystem/5(NIter) -> LocateRefNIter_Uls/1
  Demux/4 -> VqOvrRRef_Amp/1
  Demux/3 -> VdOvrRRef_Amp/1
  Demux/2 -> IqRef_Amp/1
  Demux/1 -> IdRef_Amp/1
  Switch1/1 -> Demux/1
  Mux2/1 -> Switch1/3
  VmaxTest_If_Else/1 -> Switch1/1
  IntermediateCalcs/1 -> F_ItoV_2/3(IntermediateCalcs), F_VoltTest_2/3(IntermediateCalcs), F_VoltTest_1/3(IntermediateCalcs), "F_ItoV_1 "/3(IntermediateCalcs), Bus Selector/1, F01_1_6_6_1_ForIteratorSubsystem/4(IntermediateCalcs)
  Mux1/1 -> VmaxTest_If_Else/3
  F01_1_6_6_1_ForIteratorSubsystem/4(VqRMid_Amp) -> Mux1/4
  F01_1_6_6_1_ForIteratorSubsystem/3(VdRMid_Amp) -> Mux1/3
  F01_1_6_6_1_ForIteratorSubsystem/2(IqMid_Amp) -> Mux1/2
  F01_1_6_6_1_ForIteratorSubsystem/1(IdMid_Amp) -> Mux1/1
  Mux/1 -> VmaxTest_If_Else/1
  IqMin_Amp/1 -> F_ItoV_2/2(IqRef_Amp), Mux2/2  "IqMin_Amp"
  IdMin_Amp/1 -> F_ItoV_2/1(IdRef_Amp), Mux2/1, F01_1_6_6_1_ForIteratorSubsystem/2(IdMin_Amp)  "IdMin_Amp"
  F_VoltTest_1/1(VoltTest_Uls) -> VmaxTest_If_Else/2  "VoltMaxTest_Uls"
  F_VoltTest_2/1(VoltTest_Uls) -> Switch1/2  "VoltMinTest_Uls"
  F_CalcIqCommand_1/2(IqRef_Amp) -> Mux/2, "F_ItoV_1 "/2(IqRef_Amp)  "IqMax_Amp"
  F_CalcIqCommand_1/1(IdRef_Amp) -> "F_ItoV_1 "/1(IdRef_Amp), Mux/1  "IdMax_Amp"
  "F_ItoV_1 "/2(VqR_Amp) -> F_VoltTest_1/2(VqR_Amp), Mux/4  "VqRMax_Amp"
  "F_ItoV_1 "/1(VdR_Amp) -> F_VoltTest_1/1(VdR_Amp), Mux/3  "VdRMax_Amp"
  IdMax_Amp/1 -> F_CalcIqCommand_1/4("IdRef_Amp "), F01_1_6_6_1_ForIteratorSubsystem/1(IdMax_Amp)
  MtrTrqCmd_MtrNm/1 -> F_CalcIqCommand_1/3(MtrTrqCmd_MtrNm), F01_1_6_6_1_ForIteratorSubsystem/3(MtrTrqCmd_MtrNm)
  Bus Selector/2 -> F_CalcIqCommand_1/2(Reluctance_Henry)  "<Reluctance_Henry>"
  Bus Selector/1 -> F_CalcIqCommand_1/1(EstKe_VpRadpS)  "<EstKe_VpRadpS>"
  F_ItoV_2/2(VqR_Amp) -> F_VoltTest_2/2(VqR_Amp), Mux2/4  "VqRMin_Amp"
  F_ItoV_2/1(VdR_Amp) -> F_VoltTest_2/1(VdR_Amp), Mux2/3  "VdRMin_Amp"

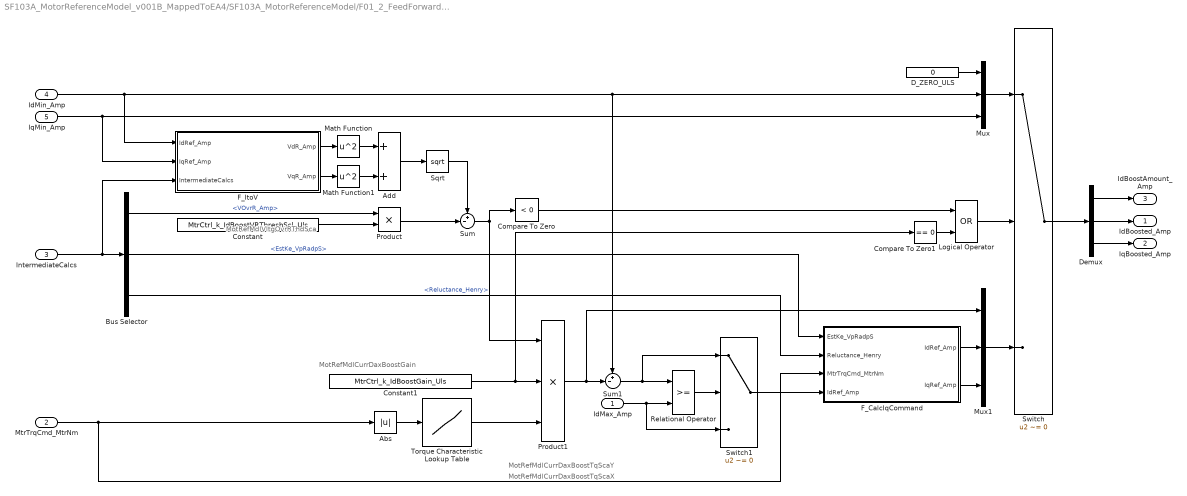
== system SF103A_MotorReferenceModel_v001B_MappedToEA4/SF103A_MotorReferenceModel/F01_2_FeedForward_Reference_Calc/F01_1_6_7_DAxisCurrentBoost ==
  note: MotRefMdlCurrDaxBoostTqScaY
  note: MotRefMdlCurrDaxBoostGain
  note: MotRefMdlCurrDaxBoostTqScaX
  note: MotRefMdlVltgOvrRThdSca
  IdMax_Amp : Inport
  MtrTrqCmd_MtrNm : Inport  Port=2
  IntermediateCalcs : Inport  Port=3
  IdMin_Amp : Inport  Port=4
  IqMin_Amp : Inport  Port=5
  Abs : Abs
  Add : Sum
  Bus Selector : BusSelector  OutputSignals=VOvrR_Amp,EstKe_VpRadpS,Reluctance_Henry
  Compare To Zero : simulink/Logic and Bit Operations/Compare To Zero  relop=<  OutDataTypeStr=uint8
  Compare To Zero1 : simulink/Logic and Bit Operations/Compare To Zero  relop===  OutDataTypeStr=uint8
  Constant : Constant  Value=MtrCtrl_k_IdBoostVRThreshScl_Uls
  Constant1 : Constant  Value=MtrCtrl_k_IdBoostGain_Uls
  D_ZERO_ULS : Constant  Value=0
  Demux : Demux  Outputs=3
  F_CalcIqCommand : Subsystem
  "F_ItoV " : Subsystem
  Logical Operator : Logic  Operator=OR  AllPortsSameDT=off  OutDataTypeStr=boolean
  Math Function : Math  Operator=square  SaturateOnIntegerOverflow=on
  Math Function1 : Math  Operator=square  SaturateOnIntegerOverflow=on
  Mux : Mux  Inputs=3
  Mux1 : Mux  Inputs=3
  Product : Product  RndMeth=Zero
  Product1 : Product  Inputs=3  RndMeth=Zero
  Relational Operator : RelationalOperator  OutDataTypeStr=boolean
  Sqrt : Sqrt  SaturateOnIntegerOverflow=on
  Sum : Sum  Inputs=+-|
  Sum1 : Sum  Inputs=+-|
  Switch : Switch  Criteria=u2 ~= 0
  Switch1 : Switch  Criteria=u2 ~= 0
  Torque Characteristic Lookup Table : Lookup  InputValues=MtrCtrl_t_IdBoostTrqCmdX_MtrNm  Table=MtrCtrl_t_IdBoostTrqCharSclY_Uls
      settings: AttributesFormatString=%<Table>\n%<InputValues>
  IdBoosted_Amp : Outport
  IqBoosted_Amp : Outport  Port=2
  IdBoostAmount_Amp : Outport  Port=3
  wires:
  Logical Operator/1 -> Switch/2
  Compare To Zero1/1 -> Logical Operator/2
  Abs/1 -> Torque Characteristic Lookup Table/1
  Math Function1/1 -> Add/2
  Math Function/1 -> Add/1
  Demux/1 -> IdBoostAmount_Amp/1
  Demux/2 -> IdBoosted_Amp/1
  Demux/3 -> IqBoosted_Amp/1
  D_ZERO_ULS/1 -> Mux/1
  F_CalcIqCommand/2(IqRef_Amp) -> Mux1/3
  Bus Selector/3 -> F_CalcIqCommand/2(Reluctance_Henry)  "<Reluctance_Henry>"
  Bus Selector/2 -> F_CalcIqCommand/1(EstKe_VpRadpS)  "<EstKe_VpRadpS>"
  Mux1/1 -> Switch/3
  F_CalcIqCommand/1(IdRef_Amp) -> Mux1/2
  Switch1/1 -> F_CalcIqCommand/4("IdRef_Amp ")
  Relational Operator/1 -> Switch1/2
  Sum1/1 -> Switch1/1, Relational Operator/1
  IdMax_Amp/1 -> Switch1/3, Relational Operator/2
  Product1/1 -> Mux1/1, Sum1/2
  Torque Characteristic Lookup Table/1 -> Product1/3
  MtrTrqCmd_MtrNm/1 -> Abs/1, F_CalcIqCommand/3(MtrTrqCmd_MtrNm)
  Constant1/1 -> Compare To Zero1/1, Product1/2
  Compare To Zero/1 -> Logical Operator/1
  Sqrt/1 -> Sum/1
  Product/1 -> Sum/2
  Add/1 -> Sqrt/1
  "F_ItoV "/1(VdR_Amp) -> Math Function/1
  Mux/1 -> Switch/1
  IqMin_Amp/1 -> Mux/3, "F_ItoV "/2(IqRef_Amp)
  IdMin_Amp/1 -> Mux/2, Sum1/1, "F_ItoV "/1(IdRef_Amp)
  Switch/1 -> Demux/1
  Sum/1 -> Product1/1, Compare To Zero/1
  Constant/1 -> Product/2
  "F_ItoV "/2(VqR_Amp) -> Math Function1/1
  Bus Selector/1 -> Product/1  "<VOvrR_Amp>"
  IntermediateCalcs/1 -> "F_ItoV "/3(IntermediateCalcs), Bus Selector/1

== system SF103A_MotorReferenceModel_v001B_MappedToEA4/SF103A_MotorReferenceModel/F01_2_FeedForward_Reference_Calc/F01_1_6_8_FeedforwardVoltage ==
  note: MODELED
  note: MODELED
  MtrVoltDaxFFStatic_Volt : Inport
  MtrVoltQaxFFStatic_Volt : Inport  Port=2
  FailOperActive_Cnt : Inport  Port=3
  MtrCurrQaxRef_Amp : Inport  Port=4
  MtrCurrDaxRef_Amp : Inport  Port=5
  IntermediateCalcs : Inport  Port=6
  EstLq_Henry : Inport  Port=7
  EstLd_Henry : Inport  Port=8
  F01_1_6_8_1_DynamicTermCalc : Subsystem
  F01_1_6_8_2_FeedforwardSelection : Subsystem
  MtrVoltDaxFF_Volt : Outport
  MtrVoltQaxFF_Volt : Outport  Port=2
  wires:
  F01_1_6_8_2_FeedforwardSelection/1(MtrVoltDaxFF_Volt) -> MtrVoltDaxFF_Volt/1
  IntermediateCalcs/1 -> F01_1_6_8_2_FeedforwardSelection/6(IntermediateCalcs)
  MtrVoltDaxFFStatic_Volt/1 -> F01_1_6_8_2_FeedforwardSelection/1(MtrVoltDaxFFStatic_Volt)
  MtrCurrDaxRef_Amp/1 -> F01_1_6_8_1_DynamicTermCalc/4(MtrCurrDaxRef_Amp)
  MtrCurrQaxRef_Amp/1 -> F01_1_6_8_1_DynamicTermCalc/3(MtrCurrQaxRef_Amp)
  F01_1_6_8_1_DynamicTermCalc/1(MtrVoltQaxFFDynTerm_Volt) -> F01_1_6_8_2_FeedforwardSelection/4(MtrVoltQaxFFDynTerm_Volt)
  F01_1_6_8_1_DynamicTermCalc/2(MtrVoltDaxFFDynTerm_Volt) -> F01_1_6_8_2_FeedforwardSelection/5(MtrVoltDaxFFDynTerm_Volt)
  FailOperActive_Cnt/1 -> F01_1_6_8_2_FeedforwardSelection/3(FailOperActive_Cnt)
  MtrVoltQaxFFStatic_Volt/1 -> F01_1_6_8_2_FeedforwardSelection/2(MtrVoltQaxFFStatic_Volt)
  EstLd_Henry/1 -> F01_1_6_8_1_DynamicTermCalc/1(EstLd_Henry)
  EstLq_Henry/1 -> F01_1_6_8_1_DynamicTermCalc/2(EstLq_Henry)
  F01_1_6_8_2_FeedforwardSelection/2(MtrVoltQaxFF_Volt) -> MtrVoltQaxFF_Volt/1

== system SF103A_MotorReferenceModel_v001B_MappedToEA4/SF103A_MotorReferenceModel/F01_2_FeedForward_Reference_Calc/F01_1_6_3_LocateTorqueExtremes/F01_1_6_3_1_FillBracketArrays ==
  note: MotRefMdlCurrDaxQaxRefDelta
  note: MotRefMdlDeltaTbl? An array of phase advance interpolation points
  Bus Creator : BusCreator  Inputs=3
  Trigonometric Function : Trigonometry
  Trigonometric Function1 : Trigonometry  Operator=cos
  t_IdqRefDeltaPoints : Constant  Value=MtrCtrl_t_IdqRefDeltaPoints_Rad  SampleTime=MtrCtrl_d_Ts_slow_s
  BracketArray : Outport
  wires:
  Bus Creator/1 -> BracketArray/1
  Trigonometric Function1/1 -> Bus Creator/3  "CosDelta"
  Trigonometric Function/1 -> Bus Creator/2  "SinDelta"
  t_IdqRefDeltaPoints/1 -> Bus Creator/1, Trigonometric Function1/1, Trigonometric Function/1  "Delta"

== system SF103A_MotorReferenceModel_v001B_MappedToEA4/SF103A_MotorReferenceModel/F01_2_FeedForward_Reference_Calc/F01_1_6_3_LocateTorqueExtremes/F01_1_6_3_2_FindPeakTorques ==
  Brackets : Inport
  MtrTrqCmd_MtrNm : Inport  Port=2
  Bus Selector : BusSelector  OutputSignals=Torque
  Constant1 : Constant  Value=[1 2 3 4 5 6 7 8]
  Constant7 : Constant  Value=[1 2 3 4 5 6 7 8]
  Divide : Product  Inputs=*/
  Divide1 : Product  Inputs=*/
  MinMax : MinMax  Function=max
  MinMax1 : MinMax
  MinMax2 : MinMax  Function=max
  MinMax3 : MinMax  Function=max
  Product (2) : Product  RndMeth=Zero
  Product (2)1 : Product  RndMeth=Zero
  Rounding Function : Rounding
  Rounding Function1 : Rounding
  Saturation (1) : Saturate  UpperLimit=1  LowerLimit=0
  Saturation (1)1 : Saturate  UpperLimit=1  LowerLimit=0
  Switch : Switch
  PeakTrqIndex : Outport
  wires:
  Switch/1 -> PeakTrqIndex/1
  MinMax2/1 -> Switch/3
  Product (2)1/1 -> MinMax2/1
  Constant1/1 -> Product (2)1/2
  Rounding Function1/1 -> Product (2)1/1
  Saturation (1)1/1 -> Rounding Function1/1
  Divide1/1 -> Saturation (1)1/1
  MinMax1/1 -> Divide1/2
  MinMax3/1 -> Switch/1
  MtrTrqCmd_MtrNm/1 -> Switch/2
  Product (2)/1 -> MinMax3/1
  Constant7/1 -> Product (2)/2
  Rounding Function/1 -> Product (2)/1
  Saturation (1)/1 -> Rounding Function/1
  Divide/1 -> Saturation (1)/1
  MinMax/1 -> Divide/2
  Bus Selector/1 -> MinMax1/1, Divide1/1, MinMax/1, Divide/1  "<Torque>"
  Brackets/1 -> Bus Selector/1

== system SF103A_MotorReferenceModel_v001B_MappedToEA4/SF103A_MotorReferenceModel/F01_2_FeedForward_Reference_Calc/F01_1_6_3_LocateTorqueExtremes/F01_1_6_3_3_ChooseDeltaBrackets ==
  note: MODELED
  note: MODELED
  BracketArray : Inport
  IntermediateCalcs : Inport  Port=2
  Bus Creator : BusCreator  Inputs=2
  Bus Selector : BusSelector  OutputSignals=Delta,SinDelta,CosDelta
  F_CalculateTorque : Subsystem
  F_VSinCosToIdIq : Subsystem
  Brackets : Outport
  wires:
  Bus Creator/1 -> Brackets/1
  F_CalculateTorque/1(Torque_MtrNm) -> Bus Creator/2  "Torque"
  F_VSinCosToIdIq/1(IdIq_Amp) -> F_CalculateTorque/1(Current)
  IntermediateCalcs/1 -> F_VSinCosToIdIq/3(IntermediateCalcs), F_CalculateTorque/2(IntermediateCalcs)
  Bus Selector/3 -> F_VSinCosToIdIq/2(CosDelta)  "<CosDelta>"
  Bus Selector/2 -> F_VSinCosToIdIq/1(SinDelta)  "<SinDelta>"
  Bus Selector/1 -> Bus Creator/1  "<Delta>"
  BracketArray/1 -> Bus Selector/1

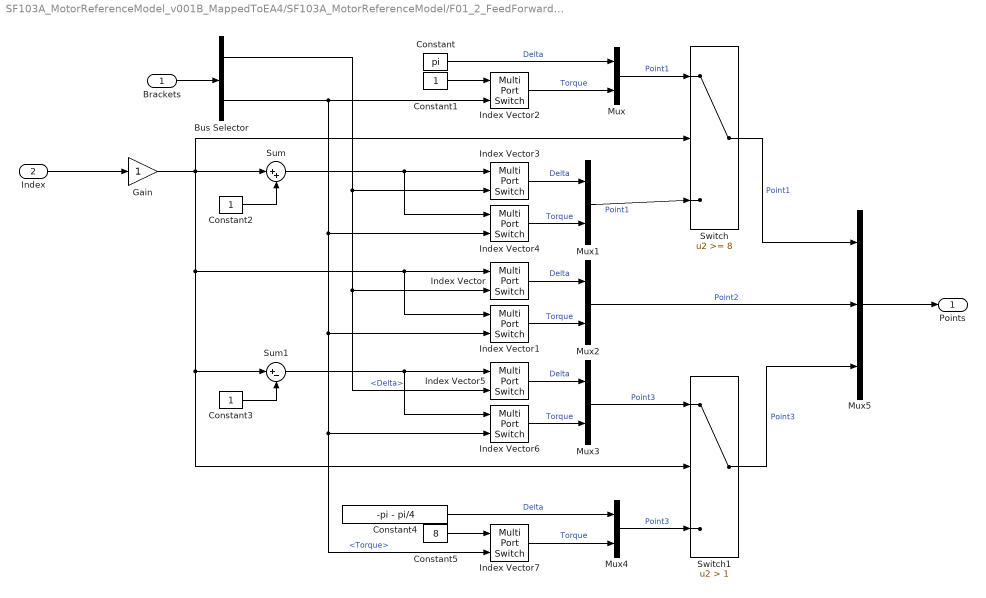
== system SF103A_MotorReferenceModel_v001B_MappedToEA4/SF103A_MotorReferenceModel/F01_2_FeedForward_Reference_Calc/F01_1_6_3_LocateTorqueExtremes/F01_1_6_3_4_WrapBracketAngles ==
  Brackets : Inport
  Index : Inport  Port=2
  Bus Selector : BusSelector  OutputSignals=Delta,Torque
  Constant : Constant  Value=pi  SampleTime=MtrCtrl_d_Ts_slow_s
  Constant1 : Constant  SampleTime=MtrCtrl_d_Ts_slow_s
  Constant2 : Constant  SampleTime=MtrCtrl_d_Ts_slow_s
  Constant3 : Constant  SampleTime=MtrCtrl_d_Ts_slow_s
  Constant4 : Constant  Value=-pi - pi/4  SampleTime=MtrCtrl_d_Ts_slow_s
  Constant5 : Constant  Value=8  SampleTime=MtrCtrl_d_Ts_slow_s
  Gain : Gain  SampleTime=MtrCtrl_d_Ts_slow_s
  Index Vector{,1..7} (8 alike) : MultiPortSwitch  Inputs=1
  Mux{,1..4} (5 alike) : Mux  Inputs=2
  Mux5 : Mux  Inputs=3
  Sum : Sum  Inputs=|++
  Sum1 : Sum  Inputs=|+-
  Switch : Switch  Threshold=8
  Switch1 : Switch  Criteria=u2 > Threshold  Threshold=1
  Points : Outport
  wires:
  Gain/1 -> Switch/2, Index Vector1/1, Index Vector/1, Switch1/2, Sum1/1, Sum/1
  Sum/1 -> Index Vector4/1, Index Vector3/1
  Mux5/1 -> Points/1
  Bus Selector/1 -> Index Vector5/2, Index Vector/2, Index Vector3/2  "<Delta>"
  Bus Selector/2 -> Index Vector7/2, Index Vector6/2, Index Vector1/2, Index Vector4/2, Index Vector2/2  "<Torque>"
  Switch1/1 -> Mux5/3  "Point3"
  Mux4/1 -> Switch1/3  "Point3"
  Index Vector7/1 -> Mux4/2  "Torque"
  Constant5/1 -> Index Vector7/1
  Constant4/1 -> Mux4/1  "Delta"
  Constant3/1 -> Sum1/2
  Sum1/1 -> Index Vector6/1, Index Vector5/1
  Mux3/1 -> Switch1/1  "Point3"
  Constant2/1 -> Sum/2
  Index Vector6/1 -> Mux3/2  "Torque"
  Index Vector5/1 -> Mux3/1  "Delta"
  Switch/1 -> Mux5/1  "Point1"
  Mux1/1 -> Switch/3  "Point1"
  Index Vector4/1 -> Mux1/2  "Torque"
  Index Vector3/1 -> Mux1/1  "Delta"
  Mux2/1 -> Mux5/2  "Point2"
  Index Vector1/1 -> Mux2/2  "Torque"
  Index Vector/1 -> Mux2/1  "Delta"
  Mux/1 -> Switch/1  "Point1"
  Index Vector2/1 -> Mux/2  "Torque"
  Constant1/1 -> Index Vector2/1
  Constant/1 -> Mux/1  "Delta"
  Index/1 -> Gain/1
  Brackets/1 -> Bus Selector/1

== system SF103A_MotorReferenceModel_v001B_MappedToEA4/SF103A_MotorReferenceModel/F01_2_FeedForward_Reference_Calc/F01_1_6_3_LocateTorqueExtremes/F01_1_6_3_5_InterpolatePeakTorque ==
  note: dMotRefMdlPkTqNrItrn
  Points : Inport
  IntermediateCalcs : Inport  Port=2
  F01_1_6_3_5_1_WhileIteratorSubsystem : Subsystem  TreatAsAtomicUnit=on
  InterPkTrqNIter_Uls : Terminator
  PeakTorque_MtrNm : Outport
  IdMax_Amp : Outport  Port=2
  PhsAdvPeak_Rad : Outport  Port=3
  wires:
  F01_1_6_3_5_1_WhileIteratorSubsystem/4(NIter) -> InterPkTrqNIter_Uls/1
  F01_1_6_3_5_1_WhileIteratorSubsystem/3(Delta_Rad) -> PhsAdvPeak_Rad/1
  F01_1_6_3_5_1_WhileIteratorSubsystem/2(IdMax_Amp) -> IdMax_Amp/1
  F01_1_6_3_5_1_WhileIteratorSubsystem/1(Torque_MtrNm) -> PeakTorque_MtrNm/1
  Points/1 -> F01_1_6_3_5_1_WhileIteratorSubsystem/2(Points)
  IntermediateCalcs/1 -> F01_1_6_3_5_1_WhileIteratorSubsystem/1(IntermediateCalcs)

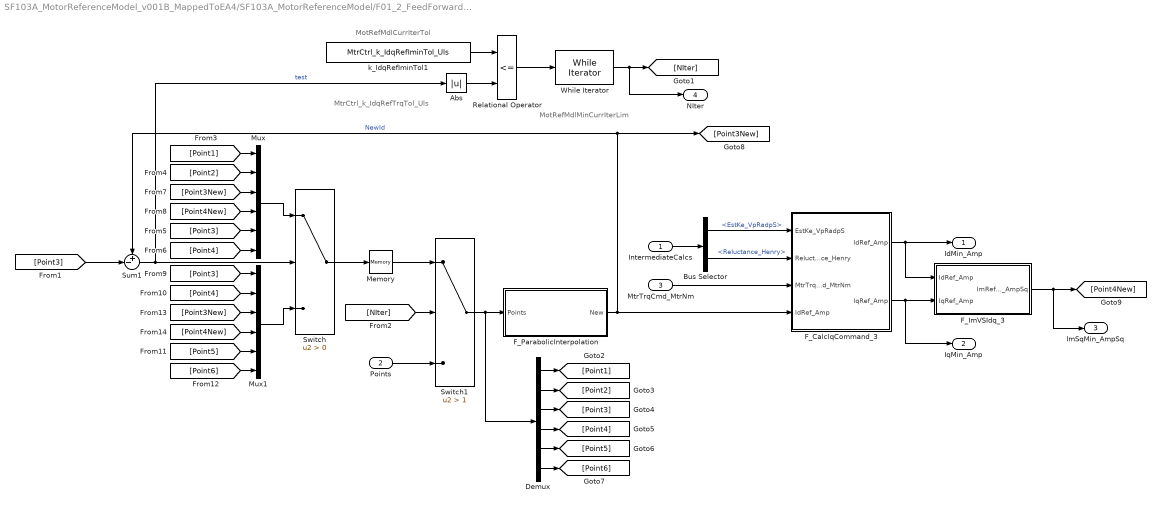
== system SF103A_MotorReferenceModel_v001B_MappedToEA4/SF103A_MotorReferenceModel/F01_2_FeedForward_Reference_Calc/F01_1_6_5_LocateMinIm/F01_1_6_5_1_WhileIteratorSubsystem ==
  note: MtrCtrl_k_IdqRefTrqTol_Uls
  note: MotRefMdlMinCurrIterLim
  note: MotRefMdlCurrIterTol
  IntermediateCalcs : Inport
  Points : Inport  Port=2
  MtrTrqCmd_MtrNm : Inport  Port=3
  Abs : Abs
  Bus Selector : BusSelector  OutputSignals=EstKe_VpRadpS,Reluctance_Henry
  Demux : Demux  Outputs=6
  F_CalcIqCommand_3 : Subsystem
  F_ImVSIdq_3 : Subsystem
  F_ParabolicInterpolation : Subsystem
  Memory : Memory  InheritSampleTime=on
  Mux : Mux  Inputs=6
  Mux1 : Mux  Inputs=6
  Relational Operator : RelationalOperator  Operator=<=  OutDataTypeStr=boolean
  Sum1 : Sum  Inputs=+-|
  Switch : Switch  Criteria=u2 > Threshold
  Switch1 : Switch  Criteria=u2 > Threshold  Threshold=1
  While Iterator : WhileIterator  MaxIters=MtrCtrl_k_IdqRefIminNIter_Uls  WhileBlockType=do-while  ShowIterationPort=on
      settings: AttributesFormatString=%<MaxIters>
  k_IdqRefIminTol1 : Constant  Value=MtrCtrl_k_IdqRefIminTol_Uls
  IdMin_Amp : Outport
  IqMin_Amp : Outport  Port=2
  ImSqMin_AmpSq : Outport  Port=3
  NIter : Outport  Port=4
  wires:
  k_IdqRefIminTol1/1 -> Relational Operator/1
  Abs/1 -> Relational Operator/2
  F_ImVSIdq_3/1(ImRefSq_AmpSq) -> ImSqMin_AmpSq/1, [Point4New]
  F_CalcIqCommand_3/2(IqRef_Amp) -> F_ImVSIdq_3/2(IqRef_Amp), IqMin_Amp/1
  F_CalcIqCommand_3/1(IdRef_Amp) -> F_ImVSIdq_3/1(IdRef_Amp), IdMin_Amp/1
  MtrTrqCmd_MtrNm/1 -> F_CalcIqCommand_3/3(MtrTrqCmd_MtrNm)
  Bus Selector/2 -> F_CalcIqCommand_3/2(Reluctance_Henry)  "<Reluctance_Henry>"
  Bus Selector/1 -> F_CalcIqCommand_3/1(EstKe_VpRadpS)  "<EstKe_VpRadpS>"
  IntermediateCalcs/1 -> Bus Selector/1
  Mux1/1 -> Switch/3
  [Point4New] -> Mux1/4
  [Point3New] -> Mux1/3
  [Point6] -> Mux1/6
  [Point5] -> Mux1/5
  [Point3] -> Mux1/1
  [Point4] -> Mux1/2
  [Point4New] -> Mux/4
  [Point3New] -> Mux/3
  [Point4] -> Mux/6
  [Point3] -> Mux/5
  [Point1] -> Mux/1
  [Point2] -> Mux/2
  [Point3] -> Sum1/2
  Demux/6 -> [Point6]
  Demux/5 -> [Point5]
  Demux/4 -> [Point4]
  Demux/3 -> [Point3]
  Demux/2 -> [Point2]
  Demux/1 -> [Point1]
  Memory/1 -> Switch1/1
  Points/1 -> Switch1/3
  [NIter] -> Switch1/2
  Switch1/1 -> F_ParabolicInterpolation/1(Points), Demux/1
  While Iterator/1 -> NIter/1, [NIter]
  Switch/1 -> Memory/1
  Mux/1 -> Switch/1
  Sum1/1 -> Abs/1, Switch/2  "test"
  F_ParabolicInterpolation/1(New) -> F_CalcIqCommand_3/4("IdRef_Amp "), Sum1/1, [Point3New]  "NewId"
  Relational Operator/1 -> While Iterator/1

== system SF103A_MotorReferenceModel_v001B_MappedToEA4/SF103A_MotorReferenceModel/F01_2_FeedForward_Reference_Calc/F01_1_6_5_LocateMinIm/F_CalcIqCommand_1 ==
  EstKe_VpRadpS : Inport
  Reluctance_Henry : Inport  Port=2
  MtrTrqCmd_MtrNm : Inport  Port=3
  "IdRef_Amp " : Inport  Port=4
  Product : Product  RndMeth=Zero
  Product1 : Product  Inputs=*/  RndMeth=Zero
  Sum : Sum  Inputs=|++
  IdRef_Amp : Outport
  IqRef_Amp : Outport  Port=2
  wires:
  Product1/1 -> IqRef_Amp/1
  MtrTrqCmd_MtrNm/1 -> Product1/1
  Sum/1 -> Product1/2
  Product/1 -> Sum/2
  EstKe_VpRadpS/1 -> Sum/1
  "IdRef_Amp "/1 -> IdRef_Amp/1, Product/2
  Reluctance_Henry/1 -> Product/1

== system SF103A_MotorReferenceModel_v001B_MappedToEA4/SF103A_MotorReferenceModel/F01_2_FeedForward_Reference_Calc/F01_1_6_5_LocateMinIm/F_CalcIqCommand_2 ==
  EstKe_VpRadpS : Inport
  Reluctance_Henry : Inport  Port=2
  MtrTrqCmd_MtrNm : Inport  Port=3
  "IdRef_Amp " : Inport  Port=4
  Product : Product  RndMeth=Zero
  Product1 : Product  Inputs=*/  RndMeth=Zero
  Sum : Sum  Inputs=|++
  IdRef_Amp : Outport
  IqRef_Amp : Outport  Port=2
  wires:
  Reluctance_Henry/1 -> Product/1
  "IdRef_Amp "/1 -> Product/2, IdRef_Amp/1
  EstKe_VpRadpS/1 -> Sum/1
  Product/1 -> Sum/2
  Sum/1 -> Product1/2
  MtrTrqCmd_MtrNm/1 -> Product1/1
  Product1/1 -> IqRef_Amp/1

== system SF103A_MotorReferenceModel_v001B_MappedToEA4/SF103A_MotorReferenceModel/F01_2_FeedForward_Reference_Calc/F01_1_6_5_LocateMinIm/F_ImVSIdq_1 ==
  IdRef_Amp : Inport
  IqRef_Amp : Inport  Port=2
  Math Function : Math  Operator=square  SaturateOnIntegerOverflow=on
  Math Function1 : Math  Operator=square  SaturateOnIntegerOverflow=on
  Sum : Sum  Inputs=|++
  ImRefSq_AmpSq : Outport
  wires:
  Sum/1 -> ImRefSq_AmpSq/1
  Math Function1/1 -> Sum/2
  Math Function/1 -> Sum/1
  IdRef_Amp/1 -> Math Function1/1
  IqRef_Amp/1 -> Math Function/1

== system SF103A_MotorReferenceModel_v001B_MappedToEA4/SF103A_MotorReferenceModel/F01_2_FeedForward_Reference_Calc/F01_1_6_5_LocateMinIm/F_ImVSIdq_2 ==
  IdRef_Amp : Inport
  IqRef_Amp : Inport  Port=2
  Math Function : Math  Operator=square  SaturateOnIntegerOverflow=on
  Math Function1 : Math  Operator=square  SaturateOnIntegerOverflow=on
  Sum : Sum  Inputs=|++
  ImRefSq_AmpSq : Outport
  wires:
  IqRef_Amp/1 -> Math Function/1
  IdRef_Amp/1 -> Math Function1/1
  Math Function/1 -> Sum/1
  Math Function1/1 -> Sum/2
  Sum/1 -> ImRefSq_AmpSq/1
